simulink model "integratorSamples"  (R2018a)
settings: Solver=VariableStepAuto  StartTime=0.0  StopTime=20  RelTol=1e-3
libraries: commfilt2 x1
settings Model: Creator=transmogrifier  LastModifiedBy=transmogrifier

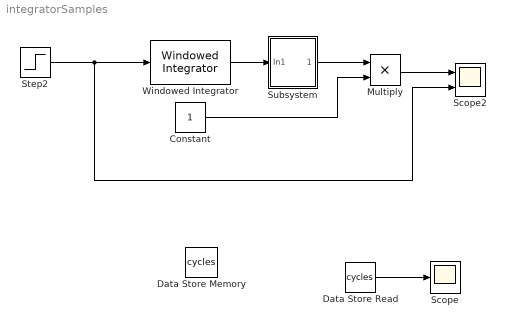
== system integratorSamples ==
  Constant : Constant
  Data Store Memory : DataStoreMemory  DataStoreName=cycles  ReadBeforeWriteMsg=warning  WriteAfterWriteMsg=warning  WriteAfterReadMsg=warning  ShowAdditionalParam=off  OutDataTypeStr=int32
  Data Store Read : DataStoreRead  DataStoreName=cycles
  Multiply : Product
  Scope : Scope
  Scope2 : Scope  NumInputPorts=2
  Step2 : Step  Time=10  SampleTime=0
  Subsystem : Subsystem
  Windowed Integrator : commfilt2/Windowed Integrator  integperiod=10  InputProcessing=Columns as channels (frame based)  roundingMode=Floor  overflowMode=off  coeffDataTypeStr=Inherit: Same word length as input  coeffMin=[]  coeffMax=[]  coeffLastDataTypeStr=Inherit: Same word length as input  accumDataTypeStr=Inherit: Same as product output  accumLastDataTypeStr=Inherit: Same as product output  outputDataTypeStr=Inherit: Same as accumulator  outputMin=[]  outputMax=[]  outputLastDataTypeStr=Inherit: Same as accumulator
      settings: SourceProductName=Communications System Toolbox  SourceProductBaseCode=CM
  wires:
  Step2/1 -> Scope2/2, Windowed Integrator/1
  Windowed Integrator/1 -> Subsystem/1(In1)
  Constant/1 -> Multiply/2
  Multiply/1 -> Scope2/1
  Subsystem/1(Out1) -> Multiply/1
  Data Store Read/1 -> Scope/1

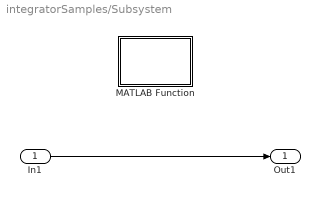
== system integratorSamples/Subsystem ==
  In1 : Inport
  MATLAB Function : MATLAB Function  TreatAsAtomicUnit=on
  Out1 : Outport
  wires:
  In1/1 -> Out1/1

== matlab function integratorSamples/Subsystem/MATLAB Function ==
  data: cycles data_store_memory
function fcn
global cycles;

cycles=cycles+1;

end
